simulink model "lab4sim"  (R2020a)
settings: Solver=VariableStepAuto  StartTime=0.0  StopTime=400  RelTol=1e-6
settings Model: Creator=ariana  LastModifiedBy=ariana

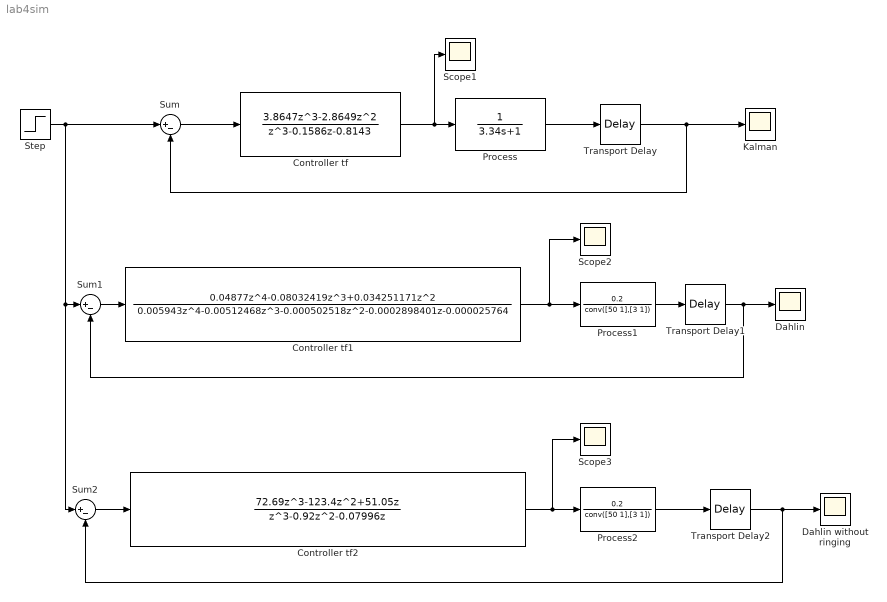
== system lab4sim ==
  " Process" : TransferFcn  Denominator=[3.34 1]
  " Process1" : TransferFcn  Numerator=[0.2]  Denominator=conv([50 1],[3 1])
  " Process2" : TransferFcn  Numerator=[0.2]  Denominator=conv([50 1],[3 1])
  Controller tf : DiscreteTransferFcn  Numerator=[3.8647 -2.8649 0 0]  Denominator=[1 0 -0.1586 -0.8143]  SampleTime=1
  Controller tf1 : DiscreteTransferFcn  Numerator=[0.04877 -0.08032419 0.034251171 0 0]  Denominator=[0.005943 -0.00512468 -0.000502518 -0.0002898401 -0.000025764]  SampleTime=1
  Controller tf2 : DiscreteTransferFcn  Numerator=[72.69 -123.4 51.05 0]  Denominator=[1 -0.92 -0.07996 0]  SampleTime=1
  Dahlin : Scope
  Dahlin without ringing : Scope
  Kalman : Scope
  Scope1 : Scope
  Scope2 : Scope
  Scope3 : Scope
  Step : Step  Time=0  SampleTime=0
  Sum : Sum  Inputs=|+-
  Sum1 : Sum  Inputs=|+-
  Sum2 : Sum  Inputs=|+-
  Transport Delay : TransportDelay  DelayTime=1.86
  Transport Delay1 : TransportDelay  DelayTime=2
  Transport Delay2 : TransportDelay  DelayTime=2
  wires:
  Step/1 -> Sum2/1, Sum1/1, Sum/1
  Sum/1 -> Controller tf/1
  Controller tf/1 -> Scope1/1, " Process"/1
  " Process"/1 -> Transport Delay/1
  Transport Delay/1 -> Sum/2, Kalman/1
  " Process1"/1 -> Transport Delay1/1
  Transport Delay1/1 -> Sum1/2, Dahlin/1
  Controller tf1/1 -> " Process1"/1, Scope2/1
  Sum1/1 -> Controller tf1/1
  Sum2/1 -> Controller tf2/1
  Controller tf2/1 -> Scope3/1, " Process2"/1
  " Process2"/1 -> Transport Delay2/1
  Transport Delay2/1 -> Sum2/2, Dahlin without ringing/1
